simulink model "System_model_discrete_2021"  (R2021a)
settings: Solver=FixedStepDiscrete  StartTime=0.0  StopTime=T_final  FixedStep=T_sample  RelTol=1e-3
values from neighbouring files (symbols this model uses):
  BDD_thresh = 0.5e-1    (= 0.05)    [run_model.m]
  C_obsv_d = C_obsv    [run_model.m]
  D_obsv_d = D_obsv    [run_model.m]
  l = n_meas    [run_model.m]
  L_obsv = place(A_bar_d.',C_obsv_d.',P).'    [run_model.m]
  load_buses = [zeros(n_gen,1); ones(n_bus-n_gen,1)]    [run_model.m]
  m = 100    [Resilient_Observer_comparison.m]    (also in run_model.m = n_meas)
  max_attack = 500    [Resilient_Observer_comparison.m]
  n = 20    [Resilient_Observer_comparison.m]    (also in run_model.m = n_states)
  n_attack = fix(m*Pa)    [Resilient_Observer_comparison.m]    (also in run_model.m = round(0.1*n_meas))
  n_bus = size(bus,1)    [run_model.m]
  n_gen = size(gen,1)    [run_model.m]
  n_meas = n_gen + n_bus    [run_model.m]
  n_states = 2*n_gen    [run_model.m]
  q0 = ones(m,T)    [run_model.m]
  Sigma = diag(sigma)    [run_model.m]
  Sigma_inv_k = diag(sigma_inv_k)    [run_model.m]
  sigma_inv_k = 1e4*(3 + 2*rand(m,1))    [run_model.m]
  size_I = n_meas - n_attack    [run_model.m]
  size_V = n_attack    [run_model.m]
  T = round(2*n)    [run_model.m]
  T_sample = 0.01    [run_model.m]
  T_start_attack = .2*T_final    (= 1.6)    [run_model.m]
  U0 = zeros(l,T)    [run_model.m]
  U_y_1 = 0    [run_model.m]
  x0 = randn(n,1)    [Resilient_Observer_comparison.m]    (also in run_model.m = zeros(n_states,1))
  Y0 = zeros(m,T)    [run_model.m]
  z_0 = zeros(n+m*T,1)    [run_model.m]
undefined symbols (not defined in the file or in its folder): A_bar_d, A_ETLO, B_bar_d, B_ETLO, G_T, HT, PhiT, Q_ETLO, r_tau, sigbuilder_block, T_start_opt, Theta_T
libraries: simulink x8
settings Model: Creator=oanubi  LastModifiedBy=Abelb
settings SolverCC: AlgebraicLoopSolver=TrustRegion
settings DebuggingCC: SFMachineParentedDataDiag=warning

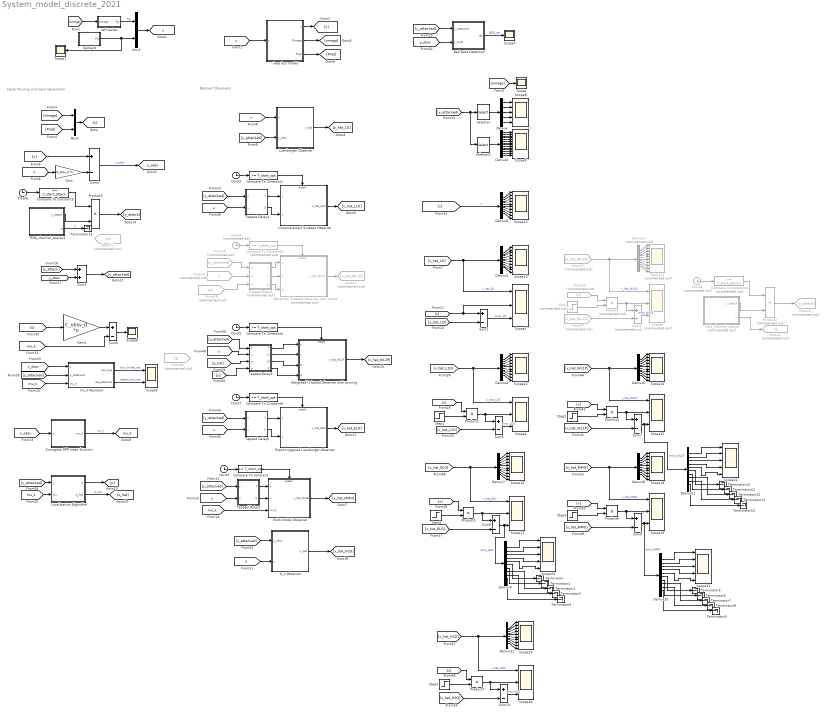
== system System_model_discrete_2021 ==
  note: Signal Routing and Input Generation
  note: Resilient Observers
  Bad Data Detection : MATLAB Function  TreatAsAtomicUnit=on
  Clock{1..2,5..7} (5 alike) : Clock
  Clock3 : Clock  Commented=on
  Clock4 : Clock  Commented=on
  Compare To Constant{,1,4,6} (4 alike) : simulink/Logic and Bit Operations/Compare To Constant  relop=>=  const=T_start_opt  OutDataTypeStr=boolean
  Compare To Constant2 : simulink/Logic and Bit Operations/Compare To Constant  Commented=on  relop=>=  const=T_start_attack  OutDataTypeStr=boolean
  Compare To Constant3 : simulink/Logic and Bit Operations/Compare To Constant  Commented=on  relop=>=  const=T_start_opt  OutDataTypeStr=boolean
  Compare To Constant5 : simulink/Logic and Bit Operations/Compare To Constant  relop=>=  const=T_start_attack  OutDataTypeStr=boolean
  Demand : Subsystem
  Demux : Demux  Outputs=n_gen
  Demux1 : Demux  Outputs=n_bus
  Demux{2,4..12} (10 alike) : Demux  Outputs=n_states
  Demux3 : Demux  Commented=on  Outputs=n_states
  Event-triggered Luenburger Observer : Subsystem
  FDIA_channel_sparse : MATLAB Function  Commented=on  TreatAsAtomicUnit=on
  FDIA_channel_sparse1 : MATLAB Function  TreatAsAtomicUnit=on
  From17 : From  Commented=on  GotoTag=x_hat_WL1O
  From18 : From  Commented=on  GotoTag=q
  From19 : From  Commented=on  GotoTag=y_attacked
  From20 : From  Commented=on  GotoTag=u  TagVisibility=global
  From22 : From  Commented=on  GotoTag=x
  From37 : From  Commented=on  GotoTag=x_hat_WL1O
  From38 : From  Commented=on  GotoTag=q
  Gain : Gain  Gain=D_obsv_d  Multiplication=Matrix(K*u) (u vector)
  Gain1 : Gain  Gain=C_obsv_d  Multiplication=Matrix(K*u) (u vector)
  Goto10 : Goto  Commented=on  GotoTag=y_attack
  Goto12 : Goto  Commented=on  GotoTag=q
  Goto13 : Goto  Commented=on  GotoTag=x_hat_WL1O
  Goto15 : Goto  Commented=on  GotoTag=q
  H_2 Observer : Subsystem
  Localization Algorithm : MATLAB Function  TreatAsAtomicUnit=on
  Luenberger Observer : Subsystem
  Multi-model Observer : Subsystem
  Mux1 : Mux  Inputs=2
  Mux2 : Mux  Inputs=2
  Product : Product  Commented=on
  Product{1,3..7} (6 alike) : Product
  Product2 : Product  Commented=on
  Scope{,2,6..7} (4 alike) : Scope
  Scope{1,4,15,17,19,24} (6 alike) : Scope  NumInputPorts=3
  Scope{10,12..14,16,18,23} (7 alike) : Scope  NumInputPorts=10
  Scope11 : Scope  Commented=on  NumInputPorts=10
  Scope{8,20..22} (4 alike) : Scope  NumInputPorts=5
  Scope3 : Scope  NumInputPorts=2
  Scope5 : Scope  Commented=on  NumInputPorts=3
  Scope9 : Scope  NumInputPorts=14
  Selector : Selector  InputPortWidth=n_meas  IndexOptions=Index vector (dialog)  Indices=1:n_gen  OutputSizes=1
  Selector1 : Selector  InputPortWidth=n_meas  IndexOptions=Index vector (dialog)  Indices=n_gen+1:n_meas  OutputSizes=1
  Step : Step  Commented=on  Time=1.5*T*T_sample  SampleTime=0
  Step{1..5} (5 alike) : Step  Time=1.5*T*T_sample  SampleTime=0
  Sum{1,3,5..10} (8 alike) : Sum  Inputs=+-
  Sum2 : Sum  Commented=on  Inputs=+-
  Sum4 : Sum
  Surrogate GPR mean function : MATLAB Function  TreatAsAtomicUnit=on
  Tapped Delay1 : Subsystem  Commented=on
  Tapped Delay2 : Subsystem
  Tapped Delay3 : Subsystem
  Tapped Delay4 : Subsystem
  Tapped Delay5 : Subsystem
  Terminator{,1..15} (16 alike) : Terminator
  Unconstrained l1-based Observer : Subsystem
  Weighted l1-based Observer with oracle : Subsystem  Commented=on
  Weighted l1-based Observer with pruning : Subsystem
  ieee bus model : Subsystem
  mu_k Residual : MATLAB Function  TreatAsAtomicUnit=on
  ref tracker : Subsystem
  tag scope: mu_k=global, u=global, y_obsv=global
  wires:
  Demux5/7 -> Scope13/7
  Selector/1 -> Demux/1
  [y_obsv] -> mu_k Residual/1(y)
  Demux/5 -> Scope8/5
  FDIA_channel_sparse/1(y_attack) -> Product2/2
  [y_attacked] -> Tapped Delay2/1(y)
  Gain/1 -> Sum5/2
  Demux2/7 -> Scope10/7
  Demand/1(Pd) -> Scope2/1, Mux1/2
  Product/1 -> Sum2/1, Scope5/2
  [y_attack] -> Sum4/1
  Demux4/4 -> Scope12/4
  Demux/4 -> Scope8/4
  Selector1/1 -> Demux1/1
  [y_obsv] -> Bad Data Detection/2(y_truth)
  Demux1/11 -> Scope9/11
  [y_obsv] -> Sum4/2
  Unconstrained l1-based Observer/1(x_hat_L1O) -> [x_hat_L1O]
  ieee bus model/2(Omega) -> [omega]
  Compare To Constant1/1 -> Unconstrained l1-based Observer/Enable
  [mu_k] -> Multi-model Observer/3(mu_k)
  Demux1/5 -> Scope9/5
  From20/1 -> Tapped Delay1/2(u)
  mu_k Residual/1(res_true) -> Scope3/1  "aux_model_res"
  Tapped Delay1/3(Q) -> Weighted l1-based Observer with oracle/3(Q)
  Demux/3 -> Scope8/3
  Weighted l1-based Observer with oracle/1(x_hat_WL1O) -> Goto13/1
  [x] -> Gain1/1
  Tapped Delay1/2(U) -> Weighted l1-based Observer with oracle/2(u)
  Tapped Delay3/2(U) -> Unconstrained l1-based Observer/2(u)
  Tapped Delay1/1(Y) -> Weighted l1-based Observer with oracle/1(y)
  Demux1/6 -> Scope9/6
  Demux3/3 -> Scope11/3
  [y_attacked] -> Tapped Delay3/1(y)
  [x_hat_L1O] -> Demux4/1, Scope4/1  "x_hat_L1O"
  FDIA_channel_sparse/2(q) -> Goto12/1
  Tapped Delay3/1(Y) -> Unconstrained l1-based Observer/1(y)
  Sum5/1 -> [y_obsv]  "y_obsv"
  From19/1 -> Tapped Delay1/1(y)
  [x] -> Product1/1
  Demux5/5 -> Scope13/5
  Demux4/2 -> Scope12/2
  Demux2/10 -> Scope10/10
  [u] -> Tapped Delay3/2(u)
  Compare To Constant3/1 -> Weighted l1-based Observer with oracle/Enable
  Sum6/1 -> Scope6/1
  Clock4/1 -> Compare To Constant3/1
  Demux5/2 -> Scope13/2
  Multi-model Observer/1(x_hat_MMO) -> [x_hat_MMO]
  Demux1/2 -> Scope9/2
  Tapped Delay2/2(U) -> Multi-model Observer/2(u)
  [omega] -> ref tracker/1(omega)
  Demux1/12 -> Scope9/12
  [x] -> Sum1/1, Scope1/2
  Demux1/8 -> Scope9/8
  Demux3/4 -> Scope11/4
  Demux5/9 -> Scope13/9
  Demux2/3 -> Scope10/3
  Sum1/1 -> Scope1/3  "error_LO"
  Demux4/6 -> Scope12/6
  From22/1 -> Product/1
  mu_k Residual/2(res_attacked) -> Scope3/2  "attack_aux_res"
  Compare To Constant2/1 -> Product2/1
  Compare To Constant/1 -> Multi-model Observer/Enable
  Demux2/5 -> Scope10/5
  Product2/1 -> Goto10/1
  Product1/1 -> Sum3/1, Scope4/2
  Demux2/1 -> Scope10/1
  [mu_k] -> Sum6/2
  Gain1/1 -> Sum6/1
  Demux3/8 -> Scope11/8
  Demux5/4 -> Scope13/4
  Clock2/1 -> Compare To Constant1/1
  [y_attacked] -> mu_k Residual/2(y_attacked)
  Demux1/9 -> Scope9/9
  Demux1/3 -> Scope9/3
  Clock1/1 -> Compare To Constant/1
  [x_hat_L1O] -> Sum3/2
  Demux1/10 -> Scope9/10
  [y] -> Sum5/1
  Step1/1 -> Product1/2
  Mux1/1 -> [u]
  Demux1/14 -> Scope9/14
  Demux/2 -> Scope8/2
  [u] -> ieee bus model/1(u)
  Demux5/6 -> Scope13/6
  [omega] -> Scope/1
  [u] -> Luenberger Observer/1(u)
  ieee bus model/1(x) -> [x]
  [y_attacked] -> Luenberger Observer/2(y_obsv)
  Sum2/1 -> Scope5/3  "error_WL10"
  Demux5/3 -> Scope13/3
  Sum3/1 -> Scope4/3  "error_L1O"
  Clock3/1 -> Compare To Constant2/1
  Demux3/7 -> Scope11/7
  Demux3/6 -> Scope11/6
  [y_obsv] -> Surrogate GPR mean function/1(y)
  Demux2/2 -> Scope10/2
  Demux4/7 -> Scope12/7
  Demux4/1 -> Scope12/1
  Sum4/1 -> [y_attacked]
  Demux4/9 -> Scope12/9
  Demux4/3 -> Scope12/3
  [mu_k] -> mu_k Residual/3(mu_k)
  [x_hat_LO] -> Sum1/2
  Demux4/5 -> Scope12/5
  Demux3/9 -> Scope11/9
  Mux2/1 -> [y]
  Demux1/7 -> Scope9/7
  Tapped Delay2/1(Y) -> Multi-model Observer/1(y)
  Demux2/8 -> Scope10/8
  [y_attacked] -> Selector1/1, Selector/1
  Step/1 -> Product/2
  Demux/1 -> Scope8/1
  Demux3/2 -> Scope11/2
  From37/1 -> Sum2/2
  [x_hat_LO] -> Demux2/1, Scope1/1  "x_hat_LO"
  Demux5/8 -> Scope13/8
  Demux1/4 -> Scope9/4
  Surrogate GPR mean function/1(mu_k) -> [mu_k]  "mu_k"
  [u] -> Tapped Delay2/2(u)
  Demux1/13 -> Scope9/13
  From17/1 -> Scope5/1, Demux3/1  "x_hat_WL1O"
  Demux2/4 -> Scope10/4
  ref tracker/1(Pg) -> Mux1/1  "Pg"
  Demux4/8 -> Scope12/8
  Demux3/5 -> Scope11/5
  Demux4/10 -> Scope12/10
  Demux3/10 -> Scope11/10
  [omega] -> Mux2/1
  Demux2/6 -> Scope10/6
  ieee bus model/3(Pnet) -> [Pnet]
  [y_attacked] -> Bad Data Detection/1(y_attacked)
  Demux5/10 -> Scope13/10
  Demux5/1 -> Scope13/1
  Demux2/9 -> Scope10/9
  Demux3/1 -> Scope11/1
  Bad Data Detection/1(res) -> Scope7/1  "BDD_res"
  Luenberger Observer/1(x_hat) -> [x_hat_LO]
  [u] -> Gain/1
  [x] -> Demux5/1  "x"
  [Pnet] -> Mux2/2
  Demux1/1 -> Scope9/1
  Clock6/1 -> Compare To Constant5/1
  Compare To Constant5/1 -> Product3/1
  FDIA_channel_sparse1/1(y_attack) -> Product3/2
  Product3/1 -> [y_attack]
  From18/1 -> Tapped Delay1/3(q)
  Tapped Delay4/3(Q) -> Weighted l1-based Observer with pruning/3(Q)
  Clock5/1 -> Compare To Constant4/1
  Tapped Delay4/2(U) -> Weighted l1-based Observer with pruning/2(u)
  Weighted l1-based Observer with pruning/1(x_hat_WL1P) -> [x_hat_WL1P]
  [y_attacked] -> Tapped Delay4/1(y)
  Tapped Delay4/1(Y) -> Weighted l1-based Observer with pruning/1(y)
  Compare To Constant4/1 -> Weighted l1-based Observer with pruning/Enable
  [u] -> Tapped Delay4/2(u)
  Demux6/1 -> Scope14/1
  Step2/1 -> Product4/2
  Demux6/5 -> Scope14/5
  Demux6/2 -> Scope14/2
  [x] -> Product4/1
  Sum7/1 -> Demux11/1, Scope15/3  "error_WL1P"
  Demux6/10 -> Scope14/10
  [x_hat_WL1P] -> Sum7/2
  [x_hat_WL1P] -> Scope15/1, Demux6/1  "x_hat_WL1P"
  Demux6/8 -> Scope14/8
  Demux6/3 -> Scope14/3
  Product4/1 -> Sum7/1, Scope15/2
  Demux6/7 -> Scope14/7
  Demux6/9 -> Scope14/9
  Demux6/4 -> Scope14/4
  Demux6/6 -> Scope14/6
  [u] -> Tapped Delay5/2(u)
  Clock7/1 -> Compare To Constant6/1
  Compare To Constant6/1 -> Event-triggered Luenburger Observer/Enable
  [y_attacked] -> Tapped Delay5/1(y)
  Tapped Delay5/2(U) -> Event-triggered Luenburger Observer/2(u)
  Tapped Delay5/1(Y) -> Event-triggered Luenburger Observer/1(y)
  Event-triggered Luenburger Observer/1(x_hat_ELO) -> [x_hat_ELO]
  Demux7/10 -> Scope16/10
  [x] -> Product5/1
  Demux7/6 -> Scope16/6
  Demux7/7 -> Scope16/7
  Demux7/3 -> Scope16/3
  Demux7/5 -> Scope16/5
  Step3/1 -> Product5/2
  [x_hat_ELO] -> Sum8/2
  Demux7/4 -> Scope16/4
  [x_hat_ELO] -> Demux7/1, Scope17/1  "x_hat_ELO"
  Product5/1 -> Sum8/1, Scope17/2
  Demux7/8 -> Scope16/8
  Sum8/1 -> Demux9/1, Scope17/3  "error_ELO"
  Demux7/2 -> Scope16/2
  Demux7/1 -> Scope16/1
  Demux7/9 -> Scope16/9
  Demux8/2 -> Scope18/2
  [x_hat_MMO] -> Scope19/1, Demux8/1  "x_hat_MMO"
  Demux8/6 -> Scope18/6
  [x] -> Product6/1
  Demux8/3 -> Scope18/3
  [x_hat_MMO] -> Sum9/2
  Demux8/4 -> Scope18/4
  Demux8/5 -> Scope18/5
  Product6/1 -> Sum9/1, Scope19/2
  Demux8/9 -> Scope18/9
  Demux8/7 -> Scope18/7
  Step4/1 -> Product6/2
  Sum9/1 -> Demux10/1, Scope19/3  "error_MMO"
  Demux8/1 -> Scope18/1
  Demux8/10 -> Scope18/10
  Demux8/8 -> Scope18/8
  Demux9/1 -> Scope20/1
  Demux9/2 -> Scope20/2
  Demux9/3 -> Scope20/3
  Demux9/4 -> Scope20/4
  Demux9/5 -> Scope20/5
  Demux9/6 -> Terminator/1
  Demux9/7 -> Terminator1/1
  Demux9/8 -> Terminator2/1
  Demux9/9 -> Terminator3/1
  Demux9/10 -> Terminator4/1
  Demux10/2 -> Scope21/2
  Demux10/3 -> Scope21/3
  Demux10/10 -> Terminator9/1
  Demux10/9 -> Terminator8/1
  Demux10/8 -> Terminator7/1
  Demux10/1 -> Scope21/1
  Demux10/7 -> Terminator6/1
  Demux10/6 -> Terminator5/1
  Demux10/5 -> Scope21/5
  Demux10/4 -> Scope21/4
  Demux11/2 -> Scope22/2
  Demux11/3 -> Scope22/3
  Demux11/10 -> Terminator14/1
  Demux11/9 -> Terminator13/1
  Demux11/8 -> Terminator12/1
  Demux11/1 -> Scope22/1
  Demux11/7 -> Terminator11/1
  Demux11/6 -> Terminator10/1
  Demux11/5 -> Scope22/5
  Demux11/4 -> Scope22/4
  [y_attacked] -> H_2 Observer/1(y_obsv)
  H_2 Observer/1(x_hat) -> [x_hat_H2O]
  [u] -> H_2 Observer/2(u)
  Demux12/4 -> Scope23/4
  Demux12/10 -> Scope23/10
  Demux12/2 -> Scope23/2
  [x_hat_H2O] -> Sum10/2
  Demux12/8 -> Scope23/8
  Step5/1 -> Product7/2
  Demux12/9 -> Scope23/9
  Demux12/3 -> Scope23/3
  Demux12/5 -> Scope23/5
  Demux12/7 -> Scope23/7
  Sum10/1 -> Scope24/3  "error_H2O"
  Product7/1 -> Sum10/1, Scope24/2
  [x] -> Product7/1
  Demux12/6 -> Scope23/6
  [x_hat_H2O] -> Demux12/1, Scope24/1  "x_hat_H2O"
  Demux12/1 -> Scope23/1
  [y_attacked] -> Localization Algorithm/1(y)
  [mu_k] -> Localization Algorithm/2(mu)
  Localization Algorithm/2(q_hat) -> [q_hat]  "q_hat"
  [q_hat] -> Tapped Delay4/3(q)
  Localization Algorithm/1(p) -> [p]
  [p] -> Tapped Delay4/4(p)
  Tapped Delay4/4(P) -> Weighted l1-based Observer with pruning/4(p)
  FDIA_channel_sparse1/2(q) -> Terminator15/1  "q"

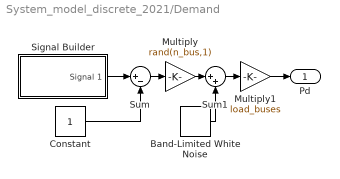
== system System_model_discrete_2021/Demand ==
  Band-Limited White Noise : simulink/Sources/Band-Limited White Noise  Cov=1e-8  Ts=0.1  seed=[23341]
  Constant : Constant
  Multiply : Gain  Gain=rand(n_bus,1)
  Multiply1 : Gain  Gain=load_buses
  Signal Builder : Subsystem  Tag=STV Subsys  LoadFcn=sigbuilder_block('load');  StartFcn=sigbuilder_block('start');  StopFcn=sigbuilder_block('stop');  ClipboardFcn=sigbuilder_block('clipboard');  mask(Sigbuilder block){tuvar=[0:10]}
      mask help: Simulink:masks:SigbuilderBlock_MD
      mask init:
      | if ~strcmp(get_param(bdroot(gcbh),'SimulationStatus'),'stopped') tuvar = sigbuilder_block('maskInit'); end
      settings: CopyFcn=sigbuilder_block('copy');  DeleteFcn=sigbuilder_block('delete');  ModelCloseFcn=sigbuilder_block('modelClose');  PreSaveFcn=sigbuilder_block('preSave');  PauseFcn=sigbuilder_block('pause');  ContinueFcn=sigbuilder_block('continue');  NameChangeFcn=sigbuilder_block('namechange');  OpenFcn=sigbuilder_block('open',[439.2 145.2 550.2 399.9 ]);  CloseFcn=sigbuilder_block('close');
      mask Display: plot(0, 0, 100, 100,[2, 2, 32, 32, 2], [68, 8, 8, 68, 68],[32, 2], [38, 38], [32, 19, 2],[53, 60, 44], [32, 17, 17, 2],[16, 16, 31, 31]);txt = getActiveGroup(gcbh);text(2, 100, txt,'verticalAlignment', 'top');
  Sum : Sum  Inputs=|+-
  Sum1 : Sum  Inputs=|++
  Pd : Outport
  wires:
  Sum/1 -> Multiply/1
  Signal Builder/1(Signal 1) -> Sum/1
  Constant/1 -> Sum/2
  Multiply/1 -> Sum1/1
  Band-Limited White Noise/1 -> Sum1/2
  Sum1/1 -> Multiply1/1
  Multiply1/1 -> Pd/1

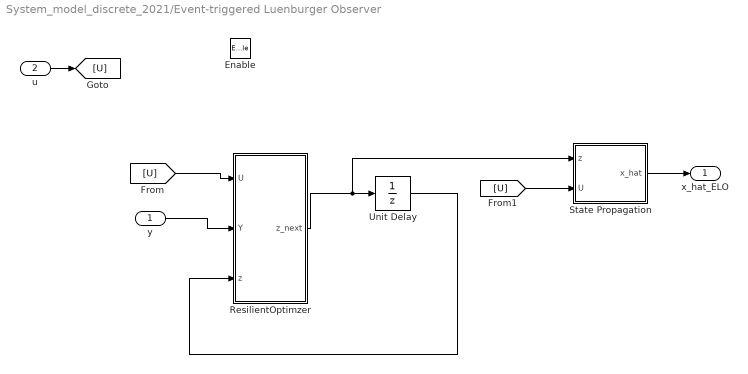
== system System_model_discrete_2021/Event-triggered Luenburger Observer ==
  y : Inport
  u : Inport  Port=2
  Enable : EnablePort
  ResilientOptimzer : MATLAB Function  TreatAsAtomicUnit=on
  State Propagation : MATLAB Function  TreatAsAtomicUnit=on
  Unit Delay : UnitDelay  InitialCondition=zeros(n_states+n_meas*T,1)  SampleTime=-1  HasFrameUpgradeWarning=on
  x_hat_ELO : Outport
  wires:
  u/1 -> [U]
  State Propagation/1(x_hat) -> x_hat_ELO/1
  [U] -> ResilientOptimzer/1(U)
  y/1 -> ResilientOptimzer/2(Y)
  ResilientOptimzer/1(z_next) -> State Propagation/1(z), Unit Delay/1
  Unit Delay/1 -> ResilientOptimzer/3(z)
  [U] -> State Propagation/2(U)

== system System_model_discrete_2021/H_2 Observer ==
  y_obsv : Inport
  u : Inport  Port=2
  Display : Display
  MATLAB Function : MATLAB Function  TreatAsAtomicUnit=on
  Unit Delay : UnitDelay  InitialCondition=zeros(n_states,1)  SampleTime=-1  HasFrameUpgradeWarning=on
  x_hat : Outport
  wires:
  MATLAB Function/1(x_next) -> Unit Delay/1
  Unit Delay/1 -> x_hat/1, MATLAB Function/1(x)
  y_obsv/1 -> MATLAB Function/2(y_obsv)
  u/1 -> MATLAB Function/3(u)
  MATLAB Function/2(P) -> Display/1

== system System_model_discrete_2021/Luenberger Observer ==
  u : Inport
  y_obsv : Inport  Port=2
  MATLAB Function : MATLAB Function  TreatAsAtomicUnit=on
  Unit Delay : UnitDelay  InitialCondition=zeros(n_states,1)  SampleTime=-1  HasFrameUpgradeWarning=on
  x_hat : Outport
  wires:
  MATLAB Function/1(x_next) -> Unit Delay/1
  Unit Delay/1 -> x_hat/1, MATLAB Function/1(x)
  u/1 -> MATLAB Function/2(u)
  y_obsv/1 -> MATLAB Function/3(y_obsv)

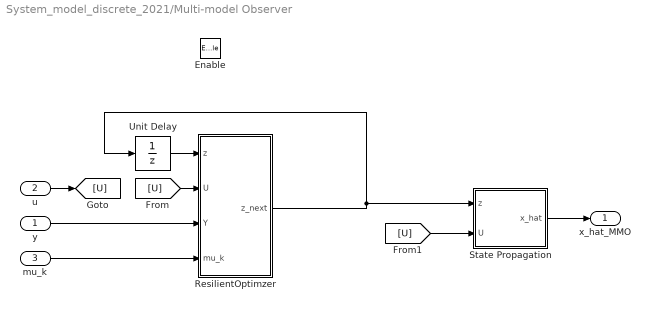
== system System_model_discrete_2021/Multi-model Observer ==
  y : Inport
  u : Inport  Port=2
  mu_k : Inport  Port=3
  Enable : EnablePort
  ResilientOptimzer : MATLAB Function  TreatAsAtomicUnit=on
  State Propagation : MATLAB Function  TreatAsAtomicUnit=on
  Unit Delay : UnitDelay  InitialCondition=z_0  SampleTime=-1  HasFrameUpgradeWarning=on
  x_hat_MMO : Outport
  wires:
  mu_k/1 -> ResilientOptimzer/4(mu_k)
  ResilientOptimzer/1(z_next) -> State Propagation/1(z), Unit Delay/1
  u/1 -> [U]
  y/1 -> ResilientOptimzer/3(Y)
  [U] -> ResilientOptimzer/2(U)
  [U] -> State Propagation/2(U)
  State Propagation/1(x_hat) -> x_hat_MMO/1
  Unit Delay/1 -> ResilientOptimzer/1(z)

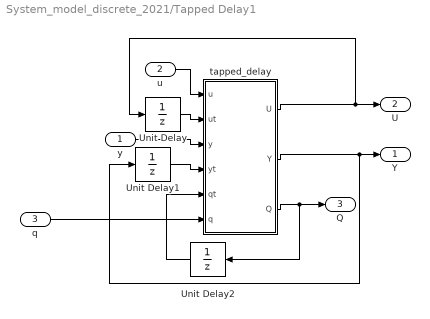
== system System_model_discrete_2021/Tapped Delay1 ==
  y : Inport
  u : Inport  Port=2
  q : Inport  Port=3
  Unit Delay : UnitDelay  InitialCondition=U0  SampleTime=-1  HasFrameUpgradeWarning=on
  Unit Delay1 : UnitDelay  InitialCondition=Y0  SampleTime=-1  HasFrameUpgradeWarning=on
  Unit Delay2 : UnitDelay  InitialCondition=q0  SampleTime=-1  HasFrameUpgradeWarning=on
  tapped_delay : MATLAB Function  TreatAsAtomicUnit=on
  Y : Outport
  U : Outport  Port=2
  Q : Outport  Port=3
  wires:
  u/1 -> tapped_delay/1(u)
  y/1 -> tapped_delay/3(y)
  tapped_delay/1(U) -> Unit Delay/1, U/1
  tapped_delay/2(Y) -> Unit Delay1/1, Y/1
  Unit Delay/1 -> tapped_delay/2(ut)
  Unit Delay1/1 -> tapped_delay/4(yt)
  tapped_delay/3(Q) -> Q/1, Unit Delay2/1
  Unit Delay2/1 -> tapped_delay/5(qt)
  q/1 -> tapped_delay/6(q)

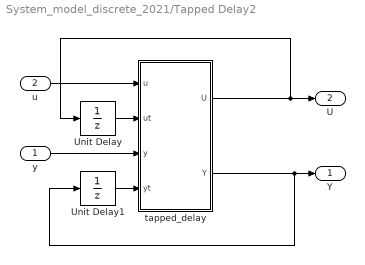
== system System_model_discrete_2021/Tapped Delay2 ==
  y : Inport
  u : Inport  Port=2
  Unit Delay : UnitDelay  InitialCondition=U0  SampleTime=-1  HasFrameUpgradeWarning=on
  Unit Delay1 : UnitDelay  InitialCondition=Y0  SampleTime=-1  HasFrameUpgradeWarning=on
  tapped_delay : MATLAB Function  TreatAsAtomicUnit=on
  Y : Outport
  U : Outport  Port=2
  wires:
  tapped_delay/2(Y) -> Y/1, Unit Delay1/1
  tapped_delay/1(U) -> U/1, Unit Delay/1
  y/1 -> tapped_delay/3(y)
  u/1 -> tapped_delay/1(u)
  Unit Delay/1 -> tapped_delay/2(ut)
  Unit Delay1/1 -> tapped_delay/4(yt)

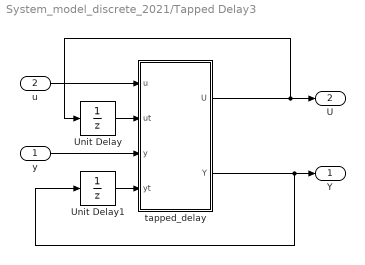
== system System_model_discrete_2021/Tapped Delay3 ==
  y : Inport
  u : Inport  Port=2
  Unit Delay : UnitDelay  InitialCondition=U0  SampleTime=-1  HasFrameUpgradeWarning=on
  Unit Delay1 : UnitDelay  InitialCondition=Y0  SampleTime=-1  HasFrameUpgradeWarning=on
  tapped_delay : MATLAB Function  TreatAsAtomicUnit=on
  Y : Outport
  U : Outport  Port=2
  wires:
  u/1 -> tapped_delay/1(u)
  y/1 -> tapped_delay/3(y)
  tapped_delay/1(U) -> Unit Delay/1, U/1
  tapped_delay/2(Y) -> Unit Delay1/1, Y/1
  Unit Delay/1 -> tapped_delay/2(ut)
  Unit Delay1/1 -> tapped_delay/4(yt)

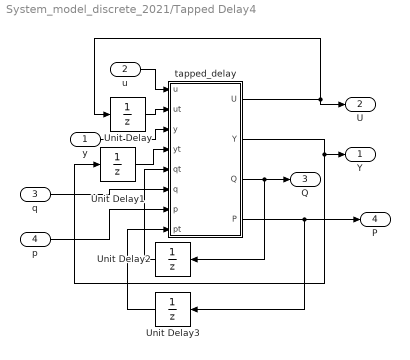
== system System_model_discrete_2021/Tapped Delay4 ==
  y : Inport
  u : Inport  Port=2
  q : Inport  Port=3
  p : Inport  Port=4
  Unit Delay : UnitDelay  InitialCondition=U0  SampleTime=-1  HasFrameUpgradeWarning=on
  Unit Delay1 : UnitDelay  InitialCondition=Y0  SampleTime=-1  HasFrameUpgradeWarning=on
  Unit Delay2 : UnitDelay  InitialCondition=q0  SampleTime=-1  HasFrameUpgradeWarning=on
  Unit Delay3 : UnitDelay  InitialCondition=q0  SampleTime=-1  HasFrameUpgradeWarning=on
  tapped_delay : MATLAB Function  TreatAsAtomicUnit=on
  Y : Outport
  U : Outport  Port=2
  Q : Outport  Port=3
  P : Outport  Port=4
  wires:
  u/1 -> tapped_delay/1(u)
  y/1 -> tapped_delay/3(y)
  tapped_delay/1(U) -> U/1, Unit Delay/1
  tapped_delay/2(Y) -> Unit Delay1/1, Y/1
  Unit Delay/1 -> tapped_delay/2(ut)
  Unit Delay1/1 -> tapped_delay/4(yt)
  tapped_delay/3(Q) -> Unit Delay2/1, Q/1
  Unit Delay2/1 -> tapped_delay/5(qt)
  q/1 -> tapped_delay/6(q)
  p/1 -> tapped_delay/7(p)
  tapped_delay/4(P) -> Unit Delay3/1, P/1
  Unit Delay3/1 -> tapped_delay/8(pt)

== system System_model_discrete_2021/Tapped Delay5 ==
  y : Inport
  u : Inport  Port=2
  Unit Delay : UnitDelay  InitialCondition=U0  SampleTime=-1  HasFrameUpgradeWarning=on
  Unit Delay1 : UnitDelay  InitialCondition=Y0  SampleTime=-1  HasFrameUpgradeWarning=on
  tapped_delay : MATLAB Function  TreatAsAtomicUnit=on
  Y : Outport
  U : Outport  Port=2
  wires:
  u/1 -> tapped_delay/1(u)
  tapped_delay/1(U) -> Unit Delay/1, U/1
  tapped_delay/2(Y) -> Unit Delay1/1, Y/1
  Unit Delay/1 -> tapped_delay/2(ut)
  Unit Delay1/1 -> tapped_delay/4(yt)
  y/1 -> tapped_delay/3(y)

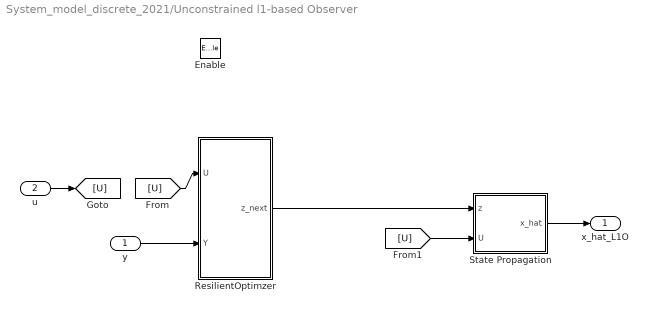
== system System_model_discrete_2021/Unconstrained l1-based Observer ==
  y : Inport
  u : Inport  Port=2
  Enable : EnablePort
  ResilientOptimzer : MATLAB Function  TreatAsAtomicUnit=on
  State Propagation : MATLAB Function  TreatAsAtomicUnit=on
  x_hat_L1O : Outport
  wires:
  ResilientOptimzer/1(z_next) -> State Propagation/1(z)
  u/1 -> [U]
  y/1 -> ResilientOptimzer/2(Y)
  [U] -> ResilientOptimzer/1(U)
  [U] -> State Propagation/2(U)
  State Propagation/1(x_hat) -> x_hat_L1O/1

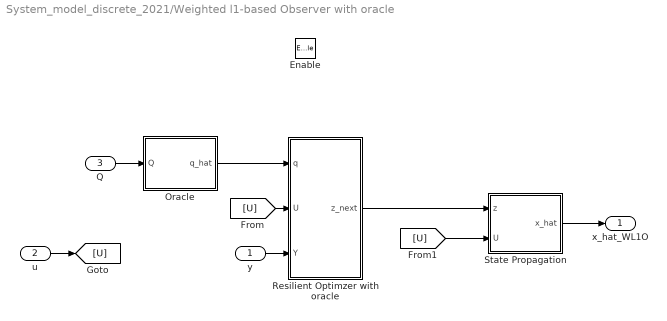
== system System_model_discrete_2021/Weighted l1-based Observer with oracle ==
  y : Inport
  u : Inport  Port=2
  Q : Inport  Port=3
  Enable : EnablePort
  Oracle : MATLAB Function  TreatAsAtomicUnit=on
  Resilient Optimzer with oracle : MATLAB Function  TreatAsAtomicUnit=on
  State Propagation : MATLAB Function  TreatAsAtomicUnit=on
  x_hat_WL1O : Outport
  wires:
  Resilient Optimzer with oracle/1(z_next) -> State Propagation/1(z)
  u/1 -> [U]
  [U] -> Resilient Optimzer with oracle/2(U)
  [U] -> State Propagation/2(U)
  State Propagation/1(x_hat) -> x_hat_WL1O/1
  Q/1 -> Oracle/1(Q)
  y/1 -> Resilient Optimzer with oracle/3(Y)
  Oracle/1(q_hat) -> Resilient Optimzer with oracle/1(q)

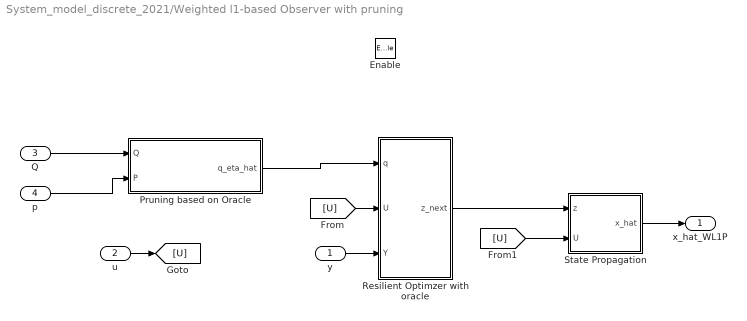
== system System_model_discrete_2021/Weighted l1-based Observer with pruning ==
  y : Inport
  u : Inport  Port=2
  Q : Inport  Port=3
  p : Inport  Port=4
  Enable : EnablePort
  Pruning based on Oracle : MATLAB Function  TreatAsAtomicUnit=on
  Resilient Optimzer with oracle : MATLAB Function  TreatAsAtomicUnit=on
  State Propagation : MATLAB Function  TreatAsAtomicUnit=on
  x_hat_WL1P : Outport
  wires:
  Resilient Optimzer with oracle/1(z_next) -> State Propagation/1(z)
  u/1 -> [U]
  [U] -> Resilient Optimzer with oracle/2(U)
  [U] -> State Propagation/2(U)
  State Propagation/1(x_hat) -> x_hat_WL1P/1
  Q/1 -> Pruning based on Oracle/1(Q)
  y/1 -> Resilient Optimzer with oracle/3(Y)
  Pruning based on Oracle/1(q_eta_hat) -> Resilient Optimzer with oracle/1(q)
  p/1 -> Pruning based on Oracle/2(P)

== system System_model_discrete_2021/ieee bus model ==
  u : Inport
  MATLAB Function : MATLAB Function  TreatAsAtomicUnit=on
  Unit Delay : UnitDelay  InitialCondition=x0  SampleTime=-1  HasFrameUpgradeWarning=on
  x : Outport
  Omega : Outport  Port=2
  Pnet : Outport  Port=3
  wires:
  MATLAB Function/1(x_next) -> Unit Delay/1
  Unit Delay/1 -> x/1, MATLAB Function/1(x)
  u/1 -> MATLAB Function/2(u)
  MATLAB Function/2(y_omega) -> Omega/1
  MATLAB Function/3(y_Pnet) -> Pnet/1

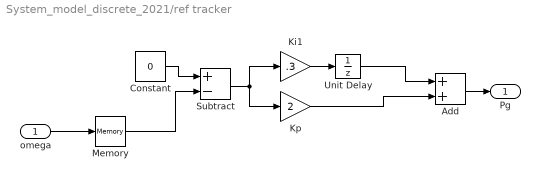
== system System_model_discrete_2021/ref tracker ==
  omega : Inport
  Add : Sum
  Constant : Constant  Value=0
  Ki1 : Gain  Gain=.3
  Kp : Gain  Gain=2
  Memory : Memory  InitialCondition=zeros(n_gen,1)
  Subtract : Sum  Inputs=+-
  Unit Delay : UnitDelay  InitialCondition=zeros(n_gen,1)  SampleTime=-1  HasFrameUpgradeWarning=on
  Pg : Outport
  wires:
  Kp/1 -> Add/2
  Unit Delay/1 -> Add/1
  Add/1 -> Pg/1
  Constant/1 -> Subtract/1
  Subtract/1 -> Ki1/1, Kp/1
  Ki1/1 -> Unit Delay/1
  Memory/1 -> Subtract/2
  omega/1 -> Memory/1

== system System_model_discrete_2021/Demand/Signal Builder ==
  Demux : Demux  Tag=STV Demux  Outputs=1
      settings: DisplayOption=none
  FromWs : FromWorkspace  Tag=STV FromWs  VariableName=tuvar
      SigBuilderData=|
      | common.afterFinalStr = 'Extrapolate'
      | common.sampleTime = 0
      | dataSet.timeRange = [0 10]
      | dataSet.name = 'Group 1'
      | sbobj.Groups.Name = 'Group 1'
      | sbobj.Groups.Signals.Name = 'Signal 1'
      | sbobj.Groups.Signals.XData = [0 0.46 1.5 2.5 4 5 6 7 10]
      | sbobj.Groups.Signals.YData = [1 1.106 1.2 1.2 0.8 0.8 1 1 1]
  Signal 1 : Outport  Tag=STV Outport
  wires:
  Demux/1 -> Signal 1/1
  FromWs/1 -> Demux/1

== matlab function System_model_discrete_2021/Multi-model Observer/State Propagation ==
  data: z input; x_hat output; U input; Theta_T parameter; G_T parameter; n parameter; T parameter; l parameter
function x_hat = fcn(z,U,Theta_T, G_T,n,T,l)
% x_hat = fcn(z,U,PhiT, HT,n_states)
% Propagates the estimated intial state to the current time
u_local = zeros(l,T-1);
u_local(:,:) = U(:,1:end-1);


% State propagation
x_hat = Theta_T*z(1:n) + G_T*u_local(:);

== matlab function System_model_discrete_2021/Unconstrained l1-based Observer/ResilientOptimzer ==
  data: z_next output; U input; Y input; HT parameter; PhiT parameter; n_states parameter; l parameter; T parameter; n_meas parameter
function z_next  = fcn(U,Y, HT, PhiT, n_states,l,T,n_meas)
u_local = zeros(l,T-1);
u_local(:,:) = U(:,1:end-1);
% vectorized
u = u_local(:);
y = Y(:);

coder.extrinsic('solver_call_unc')
z_next = zeros(n_states + n_meas*T,1);
z_next(:) = solver_call_unc(y,u,HT,PhiT);

== matlab function System_model_discrete_2021/Unconstrained l1-based Observer/State Propagation ==
  data: z input; x_hat output; U input; Theta_T parameter; G_T parameter; n parameter; T parameter; l parameter
function x_hat = fcn(z,U,Theta_T, G_T,n,T,l)
% x_hat = fcn(z,U,PhiT, HT,n_states)
% Propagates the estimated intial state to the current time
u_local = zeros(l,T-1);
u_local(:,:) = U(:,1:end-1);


% State propagation
x_hat = Theta_T*z(1:n) + G_T*u_local(:);

== matlab function System_model_discrete_2021/Tapped Delay1/tapped_delay ==
  data: u input; U output; ut input; y input; yt input; Y output; qt input; Q output; q input
function [U,Y,Q] = fcn(u,ut,y,yt,qt, q)
%% tapped_delay_array
% shift columns from tapped matrix to the left and appends most recent
% vector to the last column
%%% input
ut(:,1:end-1) = ut(:,2:end);
ut(:,end) = u;
U = ut;
%%% output
yt(:,1:end-1) = yt(:,2:end);
yt(:,end) = y;
Y = yt;
%%% attack
qt(:,1:end-1) = qt(:,2:end);
qt(:,end) = q;
Q = qt;

== matlab function System_model_discrete_2021/FDIA_channel_sparse ==
  data: n_attack parameter; y_attack output; n_meas parameter; PhiT parameter; max_attack parameter; BDD_thresh parameter; q output; T parameter
function [y_attack,q] = fcn(n_attack,n_meas,PhiT,max_attack, BDD_thresh, T)

%% Measurement Channel Attack
%  Assumptions:
%  1. The attacker knows the actual measurement
%  2. The attacker can only corrupt upto n_attack measurements
%  3. The attacker knows the BDD theshold

attack_idx = randi(n_meas,n_attack,1);
I_attack = zeros(n_attack*(T),1);

% y_attack   = gen_attack_channel(C_obsv_d, max_attack,attack_idx,0.75*BDD_thresh);
for index=1:T
    I_attack(((index-1)*n_attack+1):(index*n_attack)) = (index-1)*n_meas + attack_idx;    
end                                                       
ya = gen_attack_channel(PhiT,max_attack,I_attack,0.05); 
y_attack = ya(1:n_meas);
                                                        
q = ones(n_meas,1);
q(attack_idx) = 0;

== matlab function System_model_discrete_2021/Bad Data Detection ==
  data: y_attacked input; y_truth input; res output; U2 parameter
function res = fcn(y_attacked,y_truth,U2)

res = [norm(U2.'*y_attacked,2);
       norm(U2.'*y_truth,2)];

== matlab function System_model_discrete_2021/Tapped Delay3/tapped_delay ==
  data: u input; U output; ut input; y input; yt input; Y output
function [U,Y] = fcn(u,ut,y,yt)
%% tapped_delay_array
% shift columns from tapped matrix to the left and appends most recent
% vector to the last column
%%% input
ut(:,1:end-1) = ut(:,2:end);
ut(:,end) = u;
U = ut;
%%% output
yt(:,1:end-1) = yt(:,2:end);
yt(:,end) = y;
Y = yt;

== matlab function System_model_discrete_2021/Weighted l1-based Observer with oracle/Resilient Optimzer with oracle ==
  data: q input; z_next output; U input; Y input; HT parameter; PhiT parameter; n_states parameter; l parameter; T parameter; n_meas parameter
function z_next  = fcn(q,U,Y, HT, PhiT, n_states,l,T,n_meas)
u_local = zeros(l,T-1);
u_local(:,:) = U(:,1:end-1);
% vectorized
u = u_local(:);
y = Y(:);

coder.extrinsic('Weighted_L1_solver')
z_next = zeros(n_states + n_meas*T,1);
z_next(:) = Weighted_L1_solver(y,u,HT,PhiT,q);

== matlab function System_model_discrete_2021/Weighted l1-based Observer with oracle/State Propagation ==
  data: z input; x_hat output; U input; Theta_T parameter; G_T parameter; n parameter; T parameter; l parameter
function x_hat = fcn(z,U,Theta_T, G_T,n,T,l)
% x_hat = fcn(z,U,PhiT, HT,n_states)
% Propagates the estimated intial state to the current time
u_local = zeros(l,T-1);
u_local(:,:) = U(:,1:end-1);


% State propagation
x_hat = Theta_T*z(1:n) + G_T*u_local(:);

== matlab function System_model_discrete_2021/Weighted l1-based Observer with oracle/Oracle ==
  data: Q input; q_hat output; Tr parameter
function q_hat = fcn(Q,Tr)

q = Q(:);
N=length(q);

% perform machine learning
u = rand(N,1);
p = (0.5/(1-Tr)*u).*double(u<(1-Tr)) + (0.5 + (0.5/Tr)*(u-1+Tr)).*double(u>=(1-Tr));
epsilon = zeros(N,1);
epsilon(p>0.5) =1;                     % agreement 
q_hat = (q - (1-epsilon))./(2*epsilon-1);

== matlab function System_model_discrete_2021/FDIA_channel_sparse1 ==
  data: n_meas parameter; y_attack output; C_obsv_d parameter; max_attack parameter; BDD_thresh parameter; q output; n_attack parameter
function [y_attack,q]  = fcn(n_meas,C_obsv_d,max_attack, BDD_thresh, n_attack)

%% Measurement Channel Attack
%  Assumptions:
%  1. The attacker knows the actual measurement
%  2. The attacker can only corrupt upto n_attack measurements
%  3. The attacker knows the BDD theshold

attack_idx = randi(n_meas,n_attack,1);
y_attack   = gen_attack_channel(C_obsv_d, max_attack,attack_idx,0.75*BDD_thresh);
                                                        % NOTE THE .75
                                                        % Used
                                                        % conservatively
q = ones(n_meas,1);
q(attack_idx) = 0;

== matlab function System_model_discrete_2021/Tapped Delay4/tapped_delay ==
  data: u input; U output; ut input; y input; yt input; Y output; qt input; Q output; q input; p input; pt input; P output
function [U,Y,Q,P] = fcn(u,ut,y,yt,qt, q, p,pt)
%% tapped_delay_array
% shift columns from tapped matrix to the left and appends most recent
% vector to the last column
%%% input
ut(:,1:end-1) = ut(:,2:end);
ut(:,end) = u;
U = ut;
%%% output
yt(:,1:end-1) = yt(:,2:end);
yt(:,end) = y;
Y = yt;
%%% attack
qt(:,1:end-1) = qt(:,2:end);
qt(:,end) = q;
Q = qt;
%%% confidence
pt(:,1:end-1) = pt(:,2:end);
pt(:,end) = p;
P = pt;

== matlab function System_model_discrete_2021/Luenberger Observer/MATLAB Function ==
  data: x input; x_next output; u input; y_obsv input; L_obsv parameter; A_bar_d parameter; C_obsv_d parameter; B_bar_d parameter
function x_next  = fcn(x,u,y_obsv,L_obsv,A_bar_d,C_obsv_d,B_bar_d)
% Discrete state-space model for system

x_next = A_bar_d*x + B_bar_d*u + L_obsv*(y_obsv - C_obsv_d*x);

== matlab function System_model_discrete_2021/Weighted l1-based Observer with pruning/Pruning based on Oracle ==
  data: Q input; q_eta_hat output; P input
function q_eta_hat = fcn(Q,P)

q = Q(:);
p = P(:);
% coder.extrinsic('pruning_algorithm')

q_eta_hat = pruning_algorithm(q,p);

== matlab function System_model_discrete_2021/Weighted l1-based Observer with pruning/Resilient Optimzer with oracle ==
  data: q input; z_next output; U input; Y input; HT parameter; PhiT parameter; n_states parameter; l parameter; T parameter; n_meas parameter
function z_next  = fcn(q,U,Y, HT, PhiT, n_states,l,T,n_meas)
u_local = zeros(l,T-1);
u_local(:,:) = U(:,1:end-1);
% vectorized
u = u_local(:);
y = Y(:);

coder.extrinsic('Weighted_L1_solver')
z_next = zeros(n_states + n_meas*T,1);
z_next(:) = Weighted_L1_solver(y,u,HT,PhiT,q);

== matlab function System_model_discrete_2021/Weighted l1-based Observer with pruning/State Propagation ==
  data: z input; x_hat output; U input; Theta_T parameter; G_T parameter; n parameter; T parameter; l parameter
function x_hat = fcn(z,U,Theta_T, G_T,n,T,l)
% x_hat = fcn(z,U,PhiT, HT,n_states)
% Propagates the estimated intial state to the current time
u_local = zeros(l,T-1);
u_local(:,:) = U(:,1:end-1);


% State propagation
x_hat = Theta_T*z(1:n) + G_T*u_local(:);

== matlab function System_model_discrete_2021/Tapped Delay5/tapped_delay ==
  data: u input; U output; ut input; y input; yt input; Y output
function [U,Y] = fcn(u,ut,y,yt)
%% tapped_delay_array
% shift columns from tapped matrix to the left and appends most recent
% vector to the last column
%%% input
ut(:,1:end-1) = ut(:,2:end);
ut(:,end) = u;
U = ut;
%%% output
yt(:,1:end-1) = yt(:,2:end);
yt(:,end) = y;
Y = yt;

== matlab function System_model_discrete_2021/Event-triggered Luenburger Observer/ResilientOptimzer ==
  data: U input; Y input; A_ETLO parameter; B_ETLO parameter; z_next output; n_states parameter; T parameter; n_meas parameter; z input; Q_ETLO parameter; n_attack parameter; l parameter
function z_next   = fcn(U,Y, A_ETLO, B_ETLO,n_states,T,n_meas, z, Q_ETLO,n_attack,l)
u_local = zeros(l,T-1);
u_local(:,:) = U(:,1:end-1);
% vectorized
u = u_local(:,end);
Y = Y.';
y = Y(:);

% coder.extrinsic('solver_event_luenburger')
% z_next = zeros(n_states + n_meas*T,1);
% V = 0;

% [z_next(:), V] = solver_event_luenburger(y,u,z,A_ETLO,B_ETLO,Q_ETLO,n_attack,n_states,n_meas,T,V_last);

%% Time update
u_bar = [u;y];
z_hat = A_ETLO*z+B_ETLO*u_bar;

%% Pojection operation
z_proj = projection(z_hat,n_states,n_meas,n_attack,T);
z_next = z_proj;

%% Lyapunov-based event trigger
a = -0.01;
V = Lyapunov(y,Q_ETLO,z_proj);
sigma = 2*eye(T*n_meas);
L = Q_ETLO.' * sigma;

V_last = V;
% m1 = 0;
while V >= (1-a)*V_last
%     m2 = 0;
    z_proj = projection(z_next,n_states,n_meas,n_attack,T);
    z_hat = z_proj;
    V_temp = Lyapunov(y,Q_ETLO,z_hat);
    while V_temp >=(1-a)*V
        z_hat = z_hat + L*(y-Q_ETLO*z_hat);
        V_temp = Lyapunov(y,Q_ETLO,z_hat);
%         m2 =m2+1;
%         if m2>=2
%             break
%         end
    end
    z_next = z_hat;
%     m1 =m1+1;
%     if m1>2
%         break
%     end
end



end

function v = Lyapunov(y,Q,z)
v = 0.5 * norm(y-Q*z)^2;
end

function z_proj = projection(z,n,m,k,T)
%% function z_proj = projection(z,n,m,k,T)
% projection operator
% please refer to the Definition 4.1 in <Event-Triggered State Observers
% for Sparse Sensor Noise/Attacks>
%
% Jan.29
% Yu Zheng

e = z(n+1:end);
e_r = reshape(e,[m,T]);
e_n = vecnorm(e_r,2,2);
[~,idx] = mink(e_n,m-k);
e_r(idx,:) = 0;
e_r = e_r.';
e_proj = e_r(:);
z_proj = [z(1:n);e_proj];

end

== matlab function System_model_discrete_2021/Event-triggered Luenburger Observer/State Propagation ==
  data: z input; x_hat output; U input; Theta_T parameter; G_T parameter; n parameter; T parameter; l parameter
function x_hat = fcn(z,U,Theta_T, G_T,n,T,l)
% x_hat = fcn(z,U,PhiT, HT,n_states)
% Propagates the estimated intial state to the current time
u_local = zeros(l,T-1);
u_local(:,:) = U(:,1:end-1);


% State propagation
x_hat = Theta_T*z(1:n) + G_T*u_local(:);

== matlab function System_model_discrete_2021/Localization Algorithm ==
  data: p output; y input; q_hat output; mu input; Sigma parameter; n_meas parameter
function [p, q_hat] = fcn(y,mu,Sigma, n_meas)

%% calculate probability
z = (y - mu)./diag(Sigma);
p = 2*(ones(n_meas,1)-normcdf(abs(z)));

%% support prior and corresponding confidence
% q_hat = zeros(n_meas,1);
% q_hat(p >= 0.5) = 1;
q_hat = double(p>=0.5);

== matlab function System_model_discrete_2021/H_2 Observer/MATLAB Function ==
  data: x input; x_next output; y_obsv input; u input; A_bar_d parameter; C_obsv_d parameter; B_bar_d parameter; n_states parameter; size_V parameter; size_I parameter; L_obsv parameter; n_meas parameter; P output
function [x_next,P]  = fcn(x,y_obsv,u,A_bar_d,C_obsv_d,B_bar_d,n_states, size_V, size_I,L_obsv,n_meas)

x_hat_sum = zeros(n_states,1);
m = 0;
coder.extrinsic('local_estimate')
x_hat = zeros(n_states,1);
res = zeros(size_I,1);
F = zeros(size_I+n_states,n_states+size(B_bar_d,2));
P =zeros(size(A_bar_d));
for i = 1:size_V
    [x_hat,res,F,P]=local_estimate(size_I,n_meas,A_bar_d,C_obsv_d,B_bar_d,y_obsv,x);

    % 2-2 induced norm of A is equal to the biggest singular value of A.'*A
%     thres = svd(F.'*F);
%     thres = thres(1);
%     if norm(res) <= thres
%         x_hat_sum = x_hat+x_hat_sum;
%         m = m+1;
%     else
%         x_hat_sum = zeros(n_states,1)+x_hat_sum;
%         m = m+0;
%     end
    x_hat_sum = x_hat+x_hat_sum;
    m = m+1;
end
% if m==0
%     x_next = A_bar_d*x + B_bar_d*u + L_obsv*(y_obsv - C_obsv_d*x);
% else
%     x_hat_sum = reshape(x_hat_sum,n_states,1);
%     x_next = x_hat_sum/m;
% end
x_hat_sum = reshape(x_hat_sum,n_states,1);
x_next = x_hat_sum/m;
end

== matlab function System_model_discrete_2021/ieee bus model/MATLAB Function ==
  data: x input; x_next output; u input; y_omega output; A_bar_d parameter; C_obsv_d parameter; B_bar_d parameter; D_obsv_d parameter; n_gen parameter; n_bus parameter; y_Pnet output
function [x_next,y_omega,y_Pnet] = fcn(x,u,A_bar_d,C_obsv_d,B_bar_d,D_obsv_d,n_gen, n_bus)
% Discrete state-space model for system

x_next = A_bar_d*x + B_bar_d*u;

y = C_obsv_d*x + D_obsv_d*u;

y_omega = y(1:n_gen);
y_Pnet = y(n_gen+1:n_bus+n_gen);

== matlab function System_model_discrete_2021/Multi-model Observer/ResilientOptimzer ==
  data: z input; z_next output; U input; Y input; mu_k input; Sigma_inv_k parameter; HT parameter; PhiT parameter; r_tau parameter; n_states parameter; l parameter; T parameter; n_meas parameter
function z_next  = fcn(z,U,Y,mu_k,Sigma_inv_k, HT, PhiT, r_tau, n_states,l,T,n_meas)
u_local = zeros(l,T-1);
u_local(:,:) = U(:,1:end-1);
% vectorized
u = u_local(:);
y = Y(:);

coder.extrinsic('solver_call')
z_next = zeros(n_states + n_meas*T,1);
z_next(:) = solver_call(y,u,mu_k,Sigma_inv_k,z,HT,PhiT,r_tau);

== matlab function System_model_discrete_2021/mu_k Residual ==
  data: y input; y_attacked input; res_true output; mu_k input; Sigma_inv_k parameter; r_tau parameter; res_attacked output
function [res_true,res_attacked] = fcn(y,y_attacked,mu_k,Sigma_inv_k, r_tau)

res_true = r_tau - (y-mu_k).'*Sigma_inv_k*(y-mu_k);
res_attacked = r_tau - (y_attacked-mu_k).'*Sigma_inv_k*(y_attacked-mu_k);

== matlab function System_model_discrete_2021/Surrogate GPR mean function ==
  data: y input; mu_k output; sigma_inv_k parameter; r_tau parameter; m parameter; U_y_1 parameter
function mu_k = fcn(y,sigma_inv_k, r_tau,m,U_y_1)
% Prunes a random vector to find mu_k so that ||y-mu_k||_Sigma_inv_k <= r_tau

% first: random vector, secomd: normalize
y_rand = rand(m,1);
y_rand = sqrt(r_tau/max(sigma_inv_k))/norm(y_rand)*y_rand;

% create mu_k from y
mu_k = y - y_rand;

% mu_k = (U_y_1*U_y_1.')*y;

== matlab function System_model_discrete_2021/Tapped Delay2/tapped_delay ==
  data: u input; U output; ut input; y input; yt input; Y output
function [U,Y] = fcn(u,ut,y,yt)
%% tapped_delay_array
% shift columns from tapped matrix to the left and appends most recent
% vector to the last column
%%% input
ut(:,1:end-1) = ut(:,2:end);
ut(:,end) = u;
U = ut;
%%% output
yt(:,1:end-1) = yt(:,2:end);
yt(:,end) = y;
Y = yt;
